simulink model "Latest_Greatest_vSandberg"  (R2022b)
settings: Solver=ode4  StartTime=0  StopTime=15  FixedStep=DeltaT  RelTol=1e-6  EnableMultiTasking=on
InitFcn:
  | %run('final_report_initexternal')
  | % Bifocal Relay Mirror Spacecraft (prior to payload installation) Dynamics Simulation          TA Sands
  | clear all;close all;clc;warning off all;
  | 
  | % Simulation run parameters
  | Rate=34.3; Rate=100;  DeltaT=1/Rate;
  | 
  | % Maneuver Parameters
  | roll=0;  pitch=0; yaw=30;   roll=roll*pi/180; pitch=pitch*pi/180; yaw=yaw*pi/180;
  | SlewStart=5; SlewTime=10; SACengage=0;
  | SlewStart=5; SlewTime=5;
  | t0=SlewTime;
  | tf=SlewTime+5;
  | %%
  | 
  | %Constants0
  | Re=6371.2e3;mu=398601.2e9;          %earth radius and universal gravitation constant
  | 
  | % tht=0.5*((sin(pi/SlewTime*(u(4)+2.5)))+1).*[u(1) u(2) u(3)]';
  | % w=(30/77.1239)*0.5*(pi/SlewTime)*((cos(pi/SlewTime*(u(4)+2.5)))+1).*[u(1) u(2) u(3)]'
  | % wdot=-(30/77.1239)*0.5*(pi/SlewTime)^(2)*((sin(pi/SlewTime*(u(4)+2.5)))).*[u(1) u(2) u(3)]'
  | 
  | %compare with differentiating in real time
  | 
  | % A0=[0 0 0];
  | % tht=A0+1/2*(1-cos(pi/SlewTime*(t-SlewStart)))*(A-A0);
  | % w=1/2*(pi/SlewTime)*sin(pi/SlewTime*(t-SlewStart))*(A-A0);
  | % wdot1=1/2*(pi/SlewTime)^2*cos(pi/SlewTime*(t-SlewStart))*(A-A0);
  | 
  | %Spacecraft orbit
  | h=0;                                     %orbit altitude
  | R=Re+h;                             %orbit radius from center of earth
  | we=0.000072921158553;   %earth's angular velocity rad/solar sec(Vallado)
  | wo=sqrt(mu/(Re+h)^3);        %orbit angular velocity
  | incln=36.6001*pi/180;          %Inclination assumed Monterey Latitude
  | epsilon=12*pi/180;  alphao=0;
  | uo=0; nuo=0;                        %Start S/C beneath subsolar point
  | betasun=60; gamma=1.5;
  | a=0.545491852; b=0.314939867;  c=0.704226952;   %Assumed spacecraft rectangular size
  | Area=[b*c a*c a*b];                 %projected area~m^2 in body x,y,z directions
  | density=4.39e-14;
  | kpre=-9.9639/24/3600/180*pi*0;      %nodal precession constant assumed zero here
  | wn=kpre*(Re/(Re+h))^3.5*cos(incln); %nodal precession (zero eccentricity)
  | V=wo*(Re+h);
  | rho=asin(Re/(h+Re));                %earth angular radius
  | Cd=2.5;     psun=4.5E-6;            %Drag coefficient and solar pressure constant~N/m^2
  | Kaero=-0.5*Cd*V^2;   Psolar=2*psun;  %constants for aero and solar torque calculation
  | dL=[0.002 0.002 0.008];             %predicted distance between cp and cg
  | Kme=2.3390e-005;
  | 
  | %Spacecraft Magnetic Properties (assumed)
  | mresid=[0 0 0.01];                  %Spacecraft residual magnetic moment
  | M=mresid;                           %Magnetic unit dipole vector
  | K=7.943e15;
  | 
  | %%
  | % Determining Principal Axes Frame
  | % ACTUAL Spacecraft Inertia conditions
  | Ix=16.67;   Iy=16.67;   Iz=16.67 ;
  | Ixy=0;  Iyz=0;  Ixz=0;
  | ... (+176 lines)
StopFcn:
  | toc
  | %run('final_report_stopexternal')
  | 
  | if flag==0; Hcmg=Hcmg;else;Hcmg=HcmgMP;end;
  | Hxcmg=[];Hycmg=[];Hzcmg=[];CondA=[]; CondA_MP=[];t=[]; SingPt=[];DetA=[];
  | for i=1:max(size(A));  t=[t i*DeltaT];  H=Hcmg(:,:,i); Hx=H(1,:);  Hy=H(2,:);  Hz=H(3,:);
  | detA=det(A(:,1:3,i));Hxcmg=[Hxcmg Hx];  Hycmg=[Hycmg Hy];  Hzcmg=[Hzcmg Hz];
  | CONDA=cond(A(:,:,i));
  | DetA=[DetA detA]; DetA=1./DetA;
  | CondA=[CondA CONDA];end;   %CondA=CondA./max(CondA); DetA=DetA./max(DetA);
  | Hmag=sqrt(Hxcmg.^2+Hycmg.^2+Hzcmg.^2);x=(max(t)-DeltaT);
  | 
  | InvCondA;
  | 
  | if flag==0; MaxInvCond=min(1./CondA(10*Rate+1:end));DELTA=delta;DELTAdot=deltadot;
  | else; MaxInvCond=min(1./CondA_MP(10*Rate+1:end));DELTA=delta_MP;DELTAdot=deltadot_MP;Hcmg=HcmgMP;end;
  | %
  | ERROR=(trajectory*180/pi-Euler);
  | 
  | figure(1); wdotTrajectory=[CMDTrajectory(:,1) CMDTrajectory(:,2) CMDTrajectory(:,3)];  wTrajectory=[CMDTrajectory(:,4) CMDTrajectory(:,5) CMDTrajectory(:,6)]; ThetaTrajectory=180/pi.*[trajectory(:,1) trajectory(:,2) trajectory(:,3)]; set(gca,'fontsize',32, 'fontname','Palatino Linotype');
  | subplot(3,1,1); plot(t,wdotTrajectory, 'linewidth',2); axis tight; grid; ylabel('\omega^d^o^t_C_M_D (deg)','fontsize',32); title('Desired Angle, Rate, Acceleration Trajectories','fontsize',32);   set(gca,'XTick',0:2:15);     set(gca,'XTickLabel',{' ',' ',' ',' ',' ',' ',' ',' ','15'}); set(gca,'fontsize',32, 'fontname','Palatino Linotype');
  | subplot(3,1,2); plot(t,wTrajectory,'linewidth',2); axis tight; grid; ylabel('\omega_C_M_D (deg)','fontsize',32);set(gca,'XTick',0:2:15);     set(gca,'XTickLabel',{' ',' ',' ',' ',' ',' ',' ',' ','15'}); set(gca,'fontsize',32, 'fontname','Palatino Linotype');
  | subplot(3,1,3); plot(t,ThetaTrajectory,'linewidth',2); axis tight; grid; ylabel('\theta_C_M_D (deg)','fontsize',32); xlabel('time (sec)','fontsize',32); set(gca,'fontsize',32, 'fontname','Palatino Linotype');
  | 
  | % figure(2);
  | % subplot(2,1,1);plot(t,Hmag,'LineWidth',3);   ylabel('|H_c_m_g|','Fontsize',16);grid;axis([0,x,0,3]); set(gca,'fontsize',16);set(gca,'XTickLabel',{' ',' ',' ',' ',' ',' ',' ',' ','15'});
  | % subplot(2,1,2);plot(t,InvCondA,'linewidth',3);grid;xlabel('t(sec)','fontsize',14,'fontname','times');ylabel('Cond[A]','fontsize',14,'fontname','times');axis([0,max(t),0,21.82]); set(gca,'fontsize',16);
  | %
  | % DELTA1=DELTA(1,:);DELTA2=DELTA(2,:);DELTA3=DELTA(3,:);DELTA4=DELTA(4,:);
  | % DELTAdot1=DELTAdot(1,:);DELTAdot2=DELTAdot(2,:);DELTAdot3=DELTAdot(3,:);DELTAdot4=DELTAdot(4,:);
  | %
  | % figure(3);subplot(4,1,1);plot(t,DELTA1,'LineWidth',3); title('Gimbal Angles','fontsize',16);ylabel('\theta_1(deg)','Fontsize',14);grid;axis tight; set(gca,'XTickLabel',{' ',' ',' ',' ',' ',' ',' ',' ','15'});set(gca,'fontsize',16);
  | % subplot(4,1,2);plot(t,DELTA2,'LineWidth',3); ylabel('\theta_2(deg)','Fontsize',16);grid;axis tight; set(gca,'XTickLabel',{' ',' ',' ',' ',' ',' ',' ',' ','15'});set(gca,'fontsize',16);
  | % subplot(4,1,3);plot(t,DELTA3,'LineWidth',3); ylabel('\theta_3(deg)','Fontsize',16);grid;axis tight; set(gca,'XTickLabel',{' ',' ',' ',' ',' ',' ',' ',' ','15'});set(gca,'fontsize',16);
  | % subplot(4,1,4);plot(t,InvCondA,'linewidth',3);grid;xlabel('t(sec)','fontsize',14,'fontname','times');ylabel('Cond[A]','fontsize',14,'fontname','times');axis([0,max(t),0,21.82]); set(gca,'fontsize',16);
  | %
  | % figure(4);subplot(4,1,1);plot(t,DELTAdot1,'LineWidth',3);  title('Gimbal Angle RATES','fontsize',16); ylabel('\theta_d_o_t_1(rad/s)','Fontsize',16);grid; axis([0,x,-pi*1.1,pi*1.1]);   set(gca,'XTickLabel',{' ',' ',' ',' ',' ',' ',' ',' ','15'});set(gca,'fontsize',16);
  | % subplot(4,1,2);plot(t,DELTAdot2,'LineWidth',3);   ylabel('\theta_d_o_t_2(rad/s)','Fontsize',16);grid;axis([0,x,-pi*1.1,pi*1.1]);   set(gca,'XTickLabel',{' ',' ',' ',' ',' ',' ',' ',' ','15'});   set(gca,'fontsize',16);
  | % subplot(4,1,3);plot(t,DELTAdot3,'LineWidth',3);   ylabel('\theta_d_o_t_3(rad/s)','Fontsize',16);grid;axis([0,x,-pi*1.1,pi*1.1]); set(gca,'XTickLabel',{' ',' ',' ',' ',' ',' ',' ',' ','15'});set(gca,'fontsize',16);
  | % subplot(4,1,4);plot(t,InvCondA,'linewidth',3);grid;xlabel('t(sec)','fontsize',14,'fontname','times');ylabel('Cond[A]','fontsize',14,'fontname','times');axis([0,max(t),0,21.82]); set(gca,'fontsize',16);
  | %
  | % figure(5);
  | % subplot(4,1,1);plot(t,Hxcmg,'linewidth',3);axis([0,x,-3.25,3.25]);grid;ylabel('h_x/|h|','fontsize',16);title('Normalized Momentum','fontsize',16);set(gca,'XTickLabel',{' ',' ',' ',' ',' ',' ',' ',' ','15'});set(gca,'fontsize',16);
  | % subplot(4,1,2);plot(t,Hycmg,'linewidth',3);axis([0,x,-3.25,3.25]);grid;ylabel('h_y/|h|','fontsize',16);set(gca,'XTickLabel',{' ',' ',' ',' ',' ',' ',' ',' ','15'});set(gca,'fontsize',16);
  | % subplot(4,1,3);plot(t,Hzcmg,'linewidth',3);axis([0,x,-3.25,3.25]);grid;ylabel('h_z/|h|','fontsize',16);  set(gca,'XTickLabel',{' ',' ',' ',' ',' ',' ',' ',' ','15'});set(gca,'fontsize',16);
  | % subplot(4,1,4);plot(t,InvCondA,'linewidth',3);grid;xlabel('t(sec)','fontsize',14,'fontname','times');ylabel('Cond[A]','fontsize',14,'fontname','times');axis([0,max(t),0,21.82]); set(gca,'fontsize',16);
  | %
  | figure(6); EulerX=Euler(:,1);EulerY=Euler(:,2);EulerZ=Euler(:,3);
  | subplot(4,1,1);plot(t,EulerX,'linewidth',3); axis([0,x,min(EulerX),max(EulerX)]);grid;ylabel('\phi(deg)','fontsize',32);title('True Euler Angles','fontsize',14);  set(gca,'XTickLabel',{' ',' ',' ',' ',' ',' ',' ',' ','15'});  set(gca,'fontsize',32, 'fontname','Palatino Linotype');
  | subplot(4,1,2);plot(t,EulerY,'linewidth',3);  axis([0,x,min(EulerY),max(EulerY)]); grid;ylabel('\theta(deg)','fontsize',32);  set(gca,'XTickLabel',{' ',' ',' ',' ',' ',' ',' ',' ','15'}); set(gca,'fontsize',32, 'fontname','Palatino Linotype');
  | subplot(4,1,3);plot(t,EulerZ,'linewidth',3);axis([0,x,min(EulerZ),max(EulerZ)]);grid;  ylabel('\psi(deg)','fontsize',32);  set(gca,'XTickLabel',{' ',' ',' ',' ',' ',' ',' ',' ','15'});  set(gca,'fontsize',32, 'fontname','Palatino Linotype');
  | subplot(4,1,4);plot(t,InvCondA,'linewidth',3);grid;xlabel('t(sec)','fontsize',32,'fontname','times');ylabel('Cond[A]','fontsize',14,'fontname','times');axis([0,max(t),0,21.82]); set(gca,'fontsize',32, 'fontname','Palatino Linotype');
  | 
  | EX=ERROR(:,1);  EY=ERROR(:,2);     EZ=ERROR(:,3);
  | MeanXerror=mean(EX); Xmean=num2str(MeanXerror); xmean=['\mu_\phi=', Xmean];
  | STDx=std(EX);Xsigma=num2str(STDx);SigmaX=['    \sigma_x=' Xsigma];  xlegend=[xmean, SigmaX];
  | MeanYerror=mean(EY); Ymean=num2str(MeanYerror); ymean=['\mu_\theta=', Ymean];
  | STDy=std(EY); Ysigma=num2str(STDy);SigmaY=['    \sigma_y=' Ysigma]; ylegend=[ymean, SigmaY];
  | MeanZerror=mean(EZ); Zmean=num2str(MeanZerror); zmean=['\mu_\psi=', Zmean];
  | STDz=std(EZ);Zsigma=num2str(STDz);SigmaZ=['    \sigma_z=' Zsigma]; zlegend=[zmean, SigmaZ];
  | ... (+113 lines)
undefined symbols (not defined in the file): magnitude, svd
libraries: vrlib x9, dspinverses x8, aerospace x5, matrix_library x4, simulink_need_slupdate x2, dspadpt3 x2
(part 4 of 4)

== system Latest_Greatest_vSandberg/CMGs/Subsystem3/Subsystem4/Subsystem3/Subsystem1 ==
  note: $[\omega_d-\lambda(\theta-\theta_d),\dot\omega_d-\lambda(\omega-\omega_d)]$
  note: $[\omega_d,\dot\omega_d]$
  note: $\tilde q$
  note: $\tilde \omega/ \dot \tilde q$
  note: $\ddot q_r$
  note: $\dot q_r$
  note: Reference Trajectory
  note: Non-Reference Trajectory
  note: $\theta$
  note: $\omega$
  note: $\omega_d$
  note: $\theta_d$
  note: $\dot\omega_d$
  q : Inport
  qdot : Inport  Port=2
  q_d : Inport  Port=3
  qdot_d : Inport  Port=4
  qdotdot_d : Inport  Port=5
  Gain1 : Gain  Gain=lambda_r
  Gain2 : Gain  Gain=lambda_r
  Manual Switch1 : ManualSwitch
  Mux1 : Mux  Inputs=2
  Mux2 : Mux  Inputs=2
  Sum : Sum  Inputs=|+-
  Sum1 : Sum  Inputs=|+-
  Sum3 : Sum  Inputs=-+|
  Sum4 : Sum  Inputs=-+|
  Out1 : Outport
  wires:
  q_d/1 -> Sum/2
  qdot/1 -> Sum1/1
  Sum1/1 -> Gain2/1
  q/1 -> Sum/1
  Mux1/1 -> Manual Switch1/1
  Sum4/1 -> Mux2/2
  Sum3/1 -> Mux2/1
  Manual Switch1/1 -> Out1/1
  Gain1/1 -> Sum3/1
  Gain2/1 -> Sum4/1
  qdotdot_d/1 -> Sum4/2, Mux1/2
  Sum/1 -> Gain1/1
  qdot_d/1 -> Mux1/1, Sum3/2, Sum1/2
  Mux2/1 -> Manual Switch1/2
